simulink model "rl_ruido"  (R2023a)
settings: Solver=VariableStepAuto  StartTime=0.0  StopTime=400  RelTol=1e-3
values from neighbouring files (symbols this model uses):
  A1 = 0.0154    [parametros.m]    (also in variables.mat)
  A2 = 5e-5    (= 5e-05)    [parametros.m]    (also in variables.mat)
  az = 0.5    [parametros.m]    (also in variables.mat)
  g = 9.8    [parametros.m]    (also in variables.mat)
  H_ini = 0    [parametros.m]    (also in variables.mat)
  H_max = 0.62    [ddpg_v1.m]    (also in parametros.m; variables.mat)
  H_star = H_max/2    (= 0.31)    [parametros.m]    (also in variables.mat)
  ro = 1000    [parametros.m]    (also in variables.mat)
libraries: simulink x2, rllib x1
settings Model: Creator=emmanuel  LastModifiedBy=empg0
settings OptimizationCC: ReuseModelBlockBuffer=off

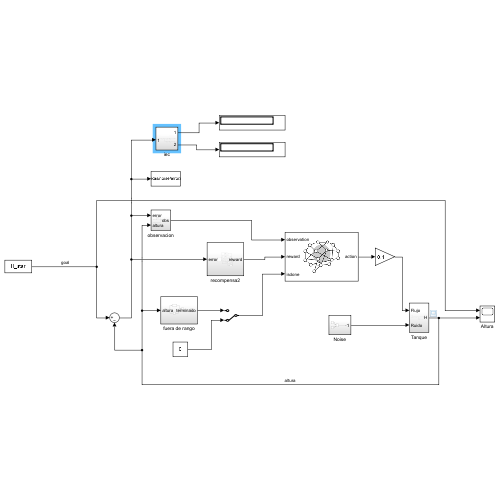
[thumbnail: Simulink's stored preview of the top-level diagram]
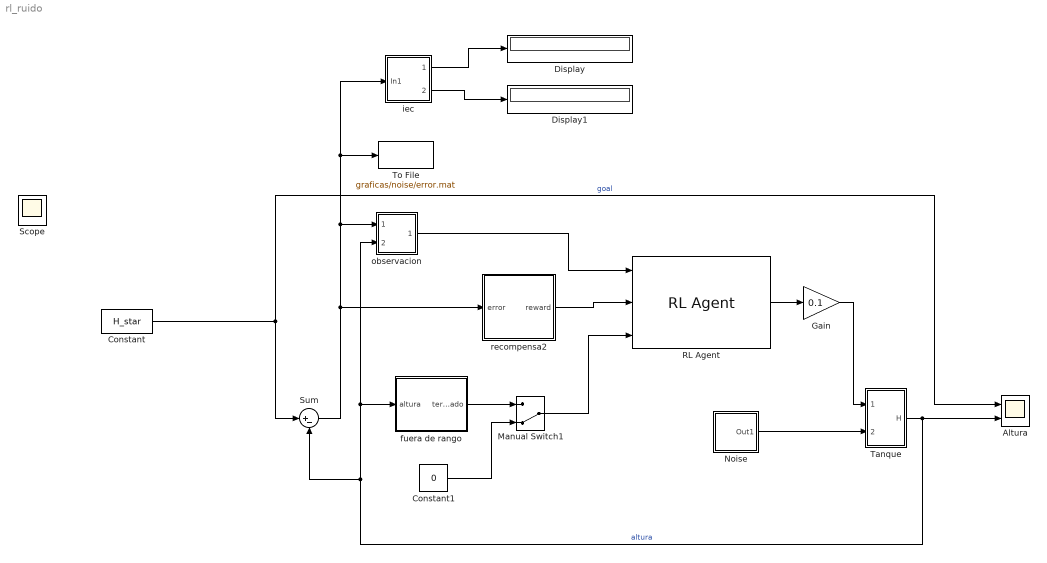
== system rl_ruido ==
  Altura : Scope  NumInputPorts=2
  Constant : Constant  Value=H_star
  Constant1 : Constant  Value=0
  Display : Display
  Display1 : Display
  Gain : Gain  Gain=0.1
  Manual Switch1 : ManualSwitch  CurrentSetting=0
  Noise : Subsystem
  RL Agent : rllib/RL Agent  Agent=agent  ExternalActionAsInput=off  ProvideLastAction=off  ProvideCumRwd=off  TreatAsDirectFeedthrough=on  UseStrictObservationDataTypes=off
  Sum : Sum  Inputs=|+-
  Tanque : Subsystem
  To File : ToFile  Filename=graficas/noise/error.mat  MatrixName=error  SampleTime=0.5
  fuera de rango : Subsystem
  iec : Subsystem
  observacion : Subsystem
  recompensa2 : Subsystem
  Scope : Scope
  wires:
  Tanque/1(H) -> fuera de rango/1(altura), observacion/2(altura), Sum/2, Altura/2  "altura"
  Sum/1 -> To File/1, iec/1(In1), observacion/1(error), recompensa2/1(error)
  observacion/1(obs) -> RL Agent/1
  fuera de rango/1(terminado) -> Manual Switch1/1
  Constant/1 -> Sum/1, Altura/1  "goal"
  Constant1/1 -> Manual Switch1/2
  Manual Switch1/1 -> RL Agent/3
  recompensa2/1(reward) -> RL Agent/2
  RL Agent/1 -> Gain/1
  Gain/1 -> Tanque/1(Flujo)
  Noise/1(Out1) -> Tanque/2(Ruido)
  iec/1(Out1) -> Display/1
  iec/2(Out2) -> Display1/1

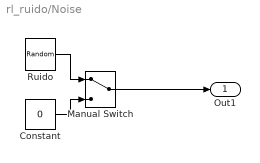
== system rl_ruido/Noise ==
  Constant : Constant  Value=0
  Manual Switch : ManualSwitch
  Ruido : UniformRandomNumber  Minimum=-0.1*0.1  Maximum=0.1*0.1  Seed=140  SampleTime=20
  Out1 : Outport
  wires:
  Ruido/1 -> Manual Switch/1
  Constant/1 -> Manual Switch/2
  Manual Switch/1 -> Out1/1

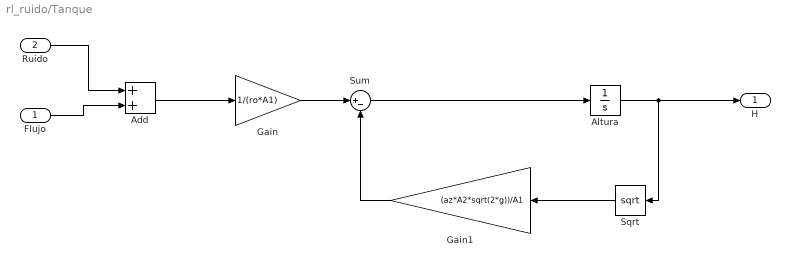
== system rl_ruido/Tanque ==
  Flujo : Inport
  Ruido : Inport  Port=2
  Add : Sum
  Altura : Integrator  InitialCondition=H_ini  LimitOutput=on  UpperSaturationLimit=0.62  LowerSaturationLimit=0
  Gain : Gain  Gain=1/(ro*A1)
  Gain1 : Gain  Gain=(az*A2*sqrt(2*g))/A1
  Sqrt : Sqrt
  Sum : Sum  Inputs=|+-
  H : Outport
  wires:
  Gain/1 -> Sum/1
  Sum/1 -> Altura/1
  Sqrt/1 -> Gain1/1
  Gain1/1 -> Sum/2
  Altura/1 -> H/1, Sqrt/1
  Add/1 -> Gain/1
  Flujo/1 -> Add/2
  Ruido/1 -> Add/1

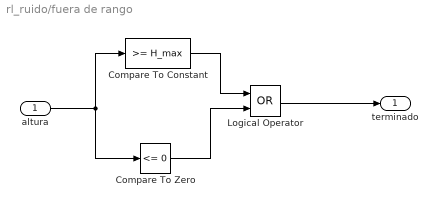
== system rl_ruido/fuera de rango ==
  altura : Inport
  Compare To Constant : simulink/Logic and Bit Operations/Compare To Constant  relop=>=  const=H_max  OutDataTypeStr=boolean
  Compare To Zero : simulink/Logic and Bit Operations/Compare To Zero  relop=<=  OutDataTypeStr=boolean
  Logical Operator : Logic  Operator=OR  AllPortsSameDT=off  OutDataTypeStr=boolean
  terminado : Outport
  wires:
  altura/1 -> Compare To Zero/1, Compare To Constant/1
  Compare To Constant/1 -> Logical Operator/1
  Compare To Zero/1 -> Logical Operator/2
  Logical Operator/1 -> terminado/1

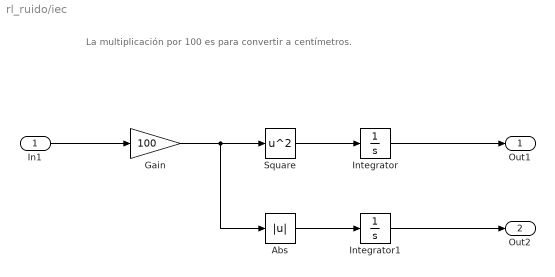
== system rl_ruido/iec ==
  note: La multiplicación por 100 es para convertir a centímetros.
  In1 : Inport
  Abs : Abs  SaturateOnIntegerOverflow=off
  Gain : Gain  Gain=100
  Integrator : Integrator
  Integrator1 : Integrator
  Square : Math  Operator=square  SignedPower=on  RndMeth=Zero
  Out1 : Outport
  Out2 : Outport  Port=2
  wires:
  Square/1 -> Integrator/1
  Integrator/1 -> Out1/1
  In1/1 -> Gain/1
  Gain/1 -> Abs/1, Square/1
  Integrator1/1 -> Out2/1
  Abs/1 -> Integrator1/1

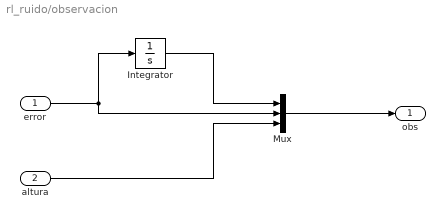
== system rl_ruido/observacion ==
  error : Inport
  altura : Inport  Port=2
  Integrator : Integrator
  Mux : Mux  Inputs=3
  obs : Outport
  wires:
  Integrator/1 -> Mux/1
  error/1 -> Integrator/1, Mux/2
  Mux/1 -> obs/1
  altura/1 -> Mux/3

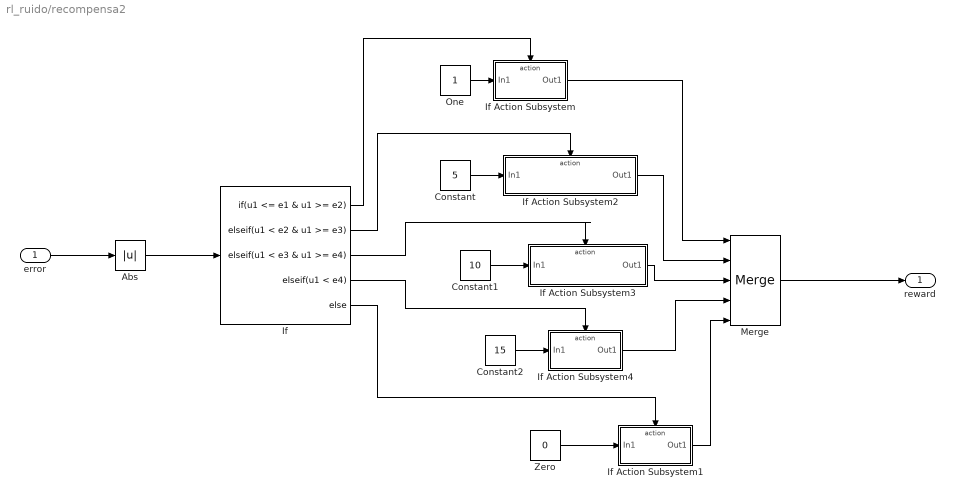
== system rl_ruido/recompensa2 ==
  error : Inport
  Abs : Abs  SaturateOnIntegerOverflow=off
  Constant : Constant  Value=5
  Constant1 : Constant  Value=10
  Constant2 : Constant  Value=15
  If : If  IfExpression=u1 <= e1 & u1 >= e2  ElseIfExpressions=u1 < e2 & u1 >= e3, u1 < e3 & u1 >= e4, u1 < e4
  If Action Subsystem : Subsystem  TreatAsAtomicUnit=on
  If Action Subsystem1 : Subsystem  TreatAsAtomicUnit=on
  If Action Subsystem2 : Subsystem  TreatAsAtomicUnit=on
  If Action Subsystem3 : Subsystem  TreatAsAtomicUnit=on
  If Action Subsystem4 : Subsystem  TreatAsAtomicUnit=on
  Merge : Merge  Inputs=5
  One : Constant  OutDataTypeStr=Inherit: Inherit via back propagation
  Zero : Constant  Value=0  OutDataTypeStr=Inherit: Inherit via back propagation
  reward : Outport
  wires:
  Abs/1 -> If/1
  error/1 -> Abs/1
  If/1 -> If Action Subsystem/Action
  Zero/1 -> If Action Subsystem1/1(In1)
  One/1 -> If Action Subsystem/1(In1)
  Merge/1 -> reward/1
  If/2 -> If Action Subsystem2/Action
  Constant/1 -> If Action Subsystem2/1(In1)
  If/3 -> If Action Subsystem3/Action
  Constant1/1 -> If Action Subsystem3/1(In1)
  If/4 -> If Action Subsystem4/Action
  If/5 -> If Action Subsystem1/Action
  Constant2/1 -> If Action Subsystem4/1(In1)
  If Action Subsystem/1(Out1) -> Merge/1
  If Action Subsystem2/1(Out1) -> Merge/2
  If Action Subsystem3/1(Out1) -> Merge/3
  If Action Subsystem4/1(Out1) -> Merge/4
  If Action Subsystem1/1(Out1) -> Merge/5

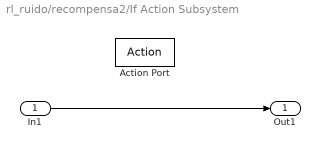
== system rl_ruido/recompensa2/If Action Subsystem ==
  In1 : Inport
  Action Port : ActionPort  ActionPortLabel=if(u1 <= e1 & u1 >= e2)
  Out1 : Outport
  wires:
  In1/1 -> Out1/1

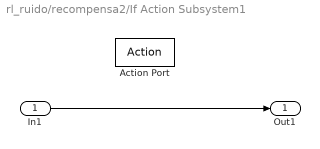
== system rl_ruido/recompensa2/If Action Subsystem1 ==
  In1 : Inport
  Action Port : ActionPort  ActionPortLabel=else
  Out1 : Outport
  wires:
  In1/1 -> Out1/1

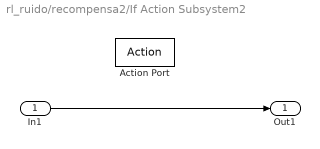
== system rl_ruido/recompensa2/If Action Subsystem2 ==
  In1 : Inport
  Action Port : ActionPort  ActionPortLabel=elseif(u1 < e2 & u1 >= e3)
  Out1 : Outport
  wires:
  In1/1 -> Out1/1

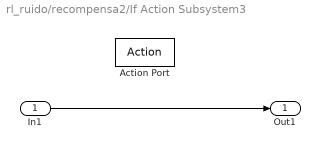
== system rl_ruido/recompensa2/If Action Subsystem3 ==
  In1 : Inport
  Action Port : ActionPort  ActionPortLabel=elseif( u1 < e3 & u1 >= e4)
  Out1 : Outport
  wires:
  In1/1 -> Out1/1

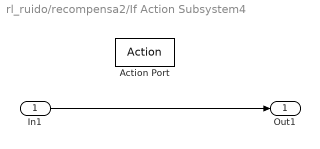
== system rl_ruido/recompensa2/If Action Subsystem4 ==
  In1 : Inport
  Action Port : ActionPort  ActionPortLabel=elseif( u1 < e4)
  Out1 : Outport
  wires:
  In1/1 -> Out1/1
